simulink model "EHB_MOTOR"  (R2023b)
settings: Solver=FixedStepDiscrete  StartTime=0.0  StopTime=inf  FixedStep=0.0001  RelTol=1e-3  EnableMultiTasking=on
undefined symbols (not defined in the file): CAN_EHB_VCU0x125, CAN_EHB_VCU0x126, CAN_id0x120_Data, Cos_Table, Cos_Table1, EHB_DTC_status, R, Sin_BreakPoint, Sin_BreakPoint1, Sin_Table, Sin_Table1, T
libraries: simulink x30
(part 1 of 9)
settings Model: Creator=dell  LastModifiedBy=17802
settings SolverCC: AlgebraicLoopSolver=TrustRegion  PositivePriorityOrder=on  AutoInsertRateTranBlk=on
settings DataIOCC: LimitDataPoints=on  ReturnWorkspaceOutputs=off
settings OptimizationCC: DefaultParameterBehavior=Inlined  UseDivisionForNetSlopeComputation=on  GainParamInheritBuiltInType=on  UseFloatMulNetSlope=on  InlineInvariantSignals=on  PassReuseOutputArgsAs=Individual arguments  ExpressionDepthLimit=2147483647  ZeroExternalMemoryAtStartup=off  ZeroInternalMemoryAtStartup=off  NoFixptDivByZeroProtection=on  EfficientFloat2IntCast=on  LifeSpan=1  MaxStackSize=64  EfficientTunableParamExpr=on
settings DebuggingCC: CheckSSInitialOutputMsg=off  UnderspecifiedInitializationDetection=Classic  MergeDetectMultiDrivingBlocksExec=none  SolverPrmCheckMsg=warning  ParameterOverflowMsg=none  ParameterPrecisionLossMsg=none  FcnCallInpInsideContextMsg=warning  UnconnectedInputMsg=warning  UnconnectedOutputMsg=warning  UnconnectedLineMsg=warning  AssertControl=EnableAll  StateNameClashWarn=warning  SFUnexpectedBacktrackingDiag=warning  SFNoUnconditionalDefaultTransitionDiag=warning  SFExecutionAtInitializationDiag=none  ArithmeticOperatorsInVariantConditions=warning
settings HardwareCC: ProdBitPerPointer=32  ProdBitPerSizeT=32  ProdBitPerPtrDiffT=32  ProdLargestAtomicInteger=Long  ProdLargestAtomicFloat=Double  ProdEndianess=BigEndian  ProdWordSize=32  ProdHWDeviceType=Freescale->MPC5xx  TargetLargestAtomicInteger=Long  TargetLargestAtomicFloat=Double  TargetIntDivRoundTo=Zero  TargetEndianess=BigEndian  TargetHWDeviceType=Freescale->32-bit PowerPC  ProdEqTarget=off
settings ModelReferenceCC: UpdateModelReferenceTargets=IfOutOfDate  EnableRefExpFcnMdlSchedulingChecks=on  PropagateSignalLabelsOutOfModel=off
settings SFSimCC: SimUseLocalCustomCode=off  MATLABDynamicMemAlloc=off  CustomCodeUndefinedFunction=UseInterfaceOnly
settings SFSimCC: SimCustomHeaderCode=|
  | #define MCU_IDLE_ST     0
  | #define MCU_INIT_ST     1
  | #define MCU_START_ST    2
  | #define MCU_RUN_ST      3
  | #define MCU_FAULT_ST    4
  | #define MCU_WAIT_ST     5
  | 
  | // MCU_IDLE_ST = 0;
  | // MCU_INIT_ST = 1;
  | // MCU_START_ST = 2;
  | // MCU_RUN_ST = 3;
  | // MCU_FAULT_ST = 4;
  | // MCU_WAIT_ST = 5;
settings RTWCC: Description=Embedded Coder  SystemTargetFile=ert.tlc  GenCodeOnly=on  TemplateMakefile=ert_default_tmf  RTWUseLocalCustomCode=off  RTWUseSimCustomCode=on  IncludeHyperlinkInReport=on
settings RTWCC: CustomHeaderCode=|
  | #define MCU_IDLE_ST     0
  | #define MCU_INIT_ST     1
  | #define MCU_START_ST    2
  | #define MCU_RUN_ST      3
  | #define MCU_FAULT_ST    4
  | #define MCU_WAIT_ST     5
  | 
  | // MCU_IDLE_ST = 0;
  | // MCU_INIT_ST = 1;
  | // MCU_START_ST = 2;
  | // MCU_RUN_ST = 3;
  | // MCU_FAULT_ST = 4;
  | // MCU_WAIT_ST = 5;
settings CodeAppCC: ForceParamTrailComments=on  IgnoreCustomStorageClasses=off  SimulinkDataObjDesc=on  CustomSymbolStrGlobalVar=EHB_MOTOR_$N$M  CustomSymbolStrType=$N$M  CustomSymbolStrFcn=$N$M$F  CustomSymbolStrFcnArg=EHB_MOTOR_$I$N$M  CustomSymbolStrBlkIO=EHB_MOTOR_B_$N$M  CustomSymbolStrMacro=$N$M  InsertBlockDesc=on  InternalIdentifier=Classic
settings ERTTargetCC: MultiwordLength=2048  IncludeMdlTerminateFcn=off  CombineSignalStateStructs=on  IncludeFileDelimiter=UseQuote  SupportAbsoluteTime=off  SupportComplex=off  SupportNonInlinedSFcns=on  InlinedParameterPlacement=NonHierarchical  ERTCustomFileTemplate=example_file_process.tlc  GlobalDataDefinition=InSeparateSourceFile  DataDefinitionFile=EHB_MOTOR_data.c  GlobalDataReference=InSeparateHeaderFile  ERTFilePackagingFormat=CompactWithDataFile  DataReferenceFile=EHB_MOTOR.h  ConvertIfToSwitch=off  SuppressUnreachableDefaultCases=off  IndentStyle=Allman  IndentSize=4  MemSecPackage=mpt
settings ConfigComp: CovMetricSettings=dw  CovSaveCumulativeToWorkspaceVar=on  CovSaveSingleToWorkspaceVar=on  CovExternalEMLEnable=off  CovSFcnEnable=off
settings SimscapeCC: SimscapeNormalizeSystem=off
settings ConfigurationSet: Description=SimMechanics 2G

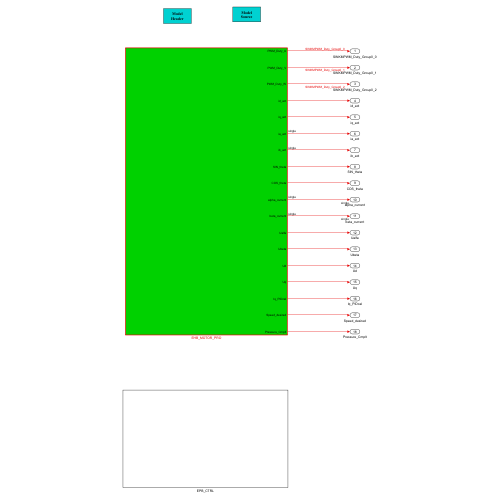
[thumbnail: Simulink's stored preview of the top-level diagram]
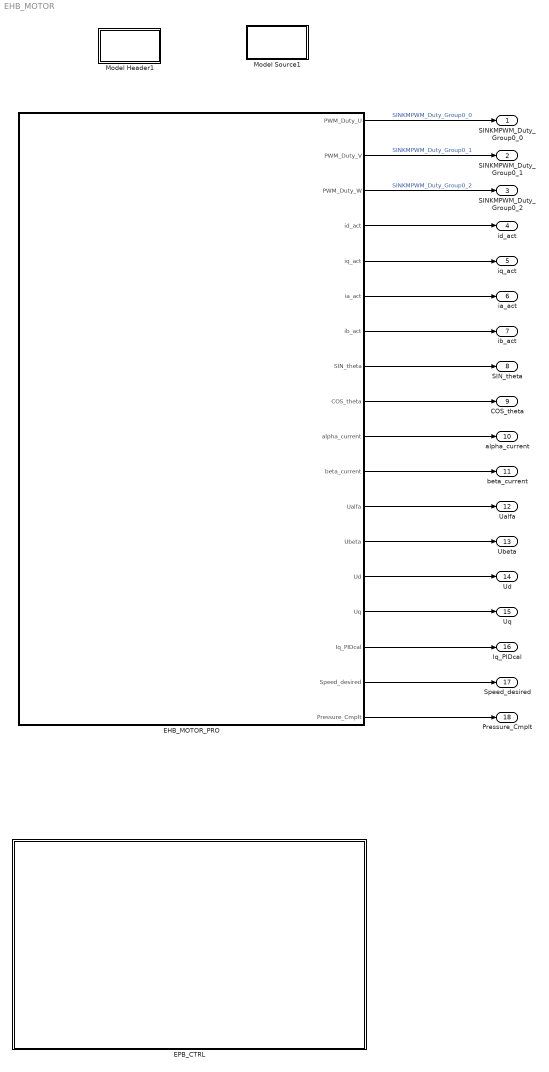
== system EHB_MOTOR ==
  EHB_MOTOR_PRO : Subsystem  TreatAsAtomicUnit=on  RTWFcnName=isr_can_rx
      settings: MinAlgLoopOccurrences=on
  EPB_CTRL : Subsystem
  Model Header1 : Subsystem  mask(Model Header){ShowInLibBrowser=0}
      mask prompts: ShowInLibBrowser "Simulink:masks:CustCodeMaskParam1_MP"
      settings: CopyFcn=cccopyfcn(gcb)  OpenFcn=ccopenfcn('Model Header')
      mask Help: eval('feval(''rtwprivate'',''rtwhelpview'',''rtw_model_header_block'')');
      mask Display: disp('Model\nHeader');
  Model Source1 : Subsystem  mask(Model Source){ShowInLibBrowser=0}
      mask prompts: ShowInLibBrowser "Simulink:masks:CustCodeMaskParam1_MP"
      settings: CopyFcn=cccopyfcn(gcb)  OpenFcn=ccopenfcn('Model Source')
      mask Help: eval('feval(''rtwprivate'',''rtwhelpview'',''rtw_model_source_block'')');
      mask Display: disp('Model\nSource');
  SINKMPWM_Duty_Group0_0 : Outport  VectorParamsAs1DForOutWhenUnconnected=off
  SINKMPWM_Duty_Group0_1 : Outport  Port=2  VectorParamsAs1DForOutWhenUnconnected=off
  SINKMPWM_Duty_Group0_2 : Outport  Port=3  VectorParamsAs1DForOutWhenUnconnected=off
  id_act : Outport  Port=4  VectorParamsAs1DForOutWhenUnconnected=off
  iq_act : Outport  Port=5  VectorParamsAs1DForOutWhenUnconnected=off
  ia_act : Outport  Port=6  VectorParamsAs1DForOutWhenUnconnected=off
  ib_act : Outport  Port=7  VectorParamsAs1DForOutWhenUnconnected=off
  SIN_theta : Outport  Port=8  VectorParamsAs1DForOutWhenUnconnected=off
  COS_theta : Outport  Port=9  VectorParamsAs1DForOutWhenUnconnected=off
  alpha_current : Outport  Port=10  OutDataTypeStr=single  VectorParamsAs1DForOutWhenUnconnected=off
  beta_current : Outport  Port=11  OutDataTypeStr=single  VectorParamsAs1DForOutWhenUnconnected=off
  Ualfa : Outport  Port=12  VectorParamsAs1DForOutWhenUnconnected=off
  Ubeta : Outport  Port=13  VectorParamsAs1DForOutWhenUnconnected=off
  Ud : Outport  Port=14  VectorParamsAs1DForOutWhenUnconnected=off
  Uq : Outport  Port=15  VectorParamsAs1DForOutWhenUnconnected=off
  Iq_PIDcal : Outport  Port=16  VectorParamsAs1DForOutWhenUnconnected=off
  Speed_desired : Outport  Port=17  VectorParamsAs1DForOutWhenUnconnected=off
  Pressure_Cmplt : Outport  Port=18  VectorParamsAs1DForOutWhenUnconnected=off
  wires:
  EHB_MOTOR_PRO/18(Pressure_Cmplt) -> Pressure_Cmplt/1
  EHB_MOTOR_PRO/4(id_act) -> id_act/1
  EHB_MOTOR_PRO/7(ib_act) -> ib_act/1
  EHB_MOTOR_PRO/16(Iq_PIDcal) -> Iq_PIDcal/1
  EHB_MOTOR_PRO/11(beta_current) -> beta_current/1
  EHB_MOTOR_PRO/15(Uq) -> Uq/1
  EHB_MOTOR_PRO/5(iq_act) -> iq_act/1
  EHB_MOTOR_PRO/13(Ubeta) -> Ubeta/1
  EHB_MOTOR_PRO/3(PWM_Duty_W) -> SINKMPWM_Duty_Group0_2/1  "SINKMPWM_Duty_Group0_2"
  EHB_MOTOR_PRO/17(Speed_desired) -> Speed_desired/1
  EHB_MOTOR_PRO/8(SIN_theta) -> SIN_theta/1
  EHB_MOTOR_PRO/6(ia_act) -> ia_act/1
  EHB_MOTOR_PRO/9(COS_theta) -> COS_theta/1
  EHB_MOTOR_PRO/14(Ud) -> Ud/1
  EHB_MOTOR_PRO/10(alpha_current) -> alpha_current/1
  EHB_MOTOR_PRO/2(PWM_Duty_V) -> SINKMPWM_Duty_Group0_1/1  "SINKMPWM_Duty_Group0_1"
  EHB_MOTOR_PRO/12(Ualfa) -> Ualfa/1
  EHB_MOTOR_PRO/1(PWM_Duty_U) -> SINKMPWM_Duty_Group0_0/1  "SINKMPWM_Duty_Group0_0"

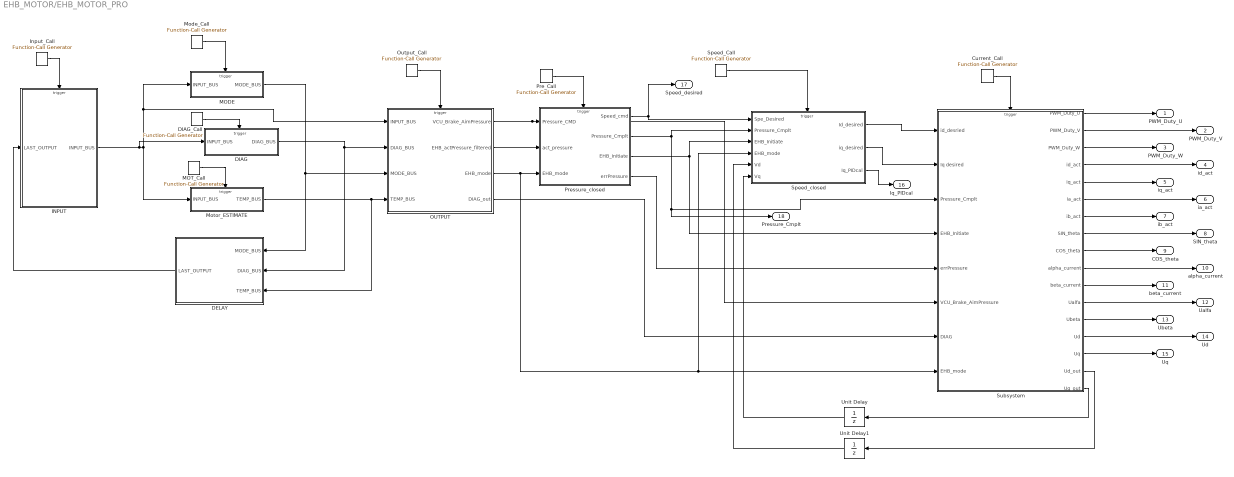
== system EHB_MOTOR/EHB_MOTOR_PRO ==
  Current_Call : simulink/Ports & Subsystems/Function-Call Generator  sample_time=0.0001  numberOfIterations=1  DisallowWideOutput=off
  DELAY : Subsystem
  DIAG : Subsystem
  DIAG_Call : simulink/Ports & Subsystems/Function-Call Generator  sample_time=0.01  numberOfIterations=1  DisallowWideOutput=off
  INPUT : Subsystem
  "Input_Call " : simulink/Ports & Subsystems/Function-Call Generator  sample_time=0.01  numberOfIterations=1  DisallowWideOutput=off
  MODE : Subsystem
  MOT_Call : simulink/Ports & Subsystems/Function-Call Generator  sample_time=0.01  numberOfIterations=1  DisallowWideOutput=off
  Mode_Call : simulink/Ports & Subsystems/Function-Call Generator  sample_time=0.01  numberOfIterations=1  DisallowWideOutput=off
  Motor_ESTIMATE : Subsystem
  OUTPUT : Subsystem
  Output_Call : simulink/Ports & Subsystems/Function-Call Generator  sample_time=0.01  numberOfIterations=1  DisallowWideOutput=off
  Pre_Call : simulink/Ports & Subsystems/Function-Call Generator  sample_time=0.002  numberOfIterations=1  DisallowWideOutput=off
  Pressure_closed : Subsystem
  "Speed_Call " : simulink/Ports & Subsystems/Function-Call Generator  sample_time=0.001  numberOfIterations=1  DisallowWideOutput=off
  Speed_closed : Subsystem
  Subsystem : Subsystem
  Unit Delay : UnitDelay  SampleTime=-1  HasFrameUpgradeWarning=on
  Unit Delay1 : UnitDelay  SampleTime=-1  HasFrameUpgradeWarning=on
  PWM_Duty_U : Outport  VectorParamsAs1DForOutWhenUnconnected=off
  PWM_Duty_V : Outport  Port=2  VectorParamsAs1DForOutWhenUnconnected=off
  PWM_Duty_W : Outport  Port=3  VectorParamsAs1DForOutWhenUnconnected=off
  id_act : Outport  Port=4  VectorParamsAs1DForOutWhenUnconnected=off
  iq_act : Outport  Port=5  VectorParamsAs1DForOutWhenUnconnected=off
  ia_act : Outport  Port=6  OutDataTypeStr=single  VectorParamsAs1DForOutWhenUnconnected=off
  ib_act : Outport  Port=7  OutDataTypeStr=single  VectorParamsAs1DForOutWhenUnconnected=off
  SIN_theta : Outport  Port=8  VectorParamsAs1DForOutWhenUnconnected=off
  COS_theta : Outport  Port=9  VectorParamsAs1DForOutWhenUnconnected=off
  alpha_current : Outport  Port=10  OutDataTypeStr=single  VectorParamsAs1DForOutWhenUnconnected=off
  beta_current : Outport  Port=11  OutDataTypeStr=single  VectorParamsAs1DForOutWhenUnconnected=off
  Ualfa : Outport  Port=12  VectorParamsAs1DForOutWhenUnconnected=off
  Ubeta : Outport  Port=13  VectorParamsAs1DForOutWhenUnconnected=off
  Ud : Outport  Port=14  VectorParamsAs1DForOutWhenUnconnected=off
  Uq : Outport  Port=15  VectorParamsAs1DForOutWhenUnconnected=off
  Iq_PIDcal : Outport  Port=16  VectorParamsAs1DForOutWhenUnconnected=off
  Speed_desired : Outport  Port=17  VectorParamsAs1DForOutWhenUnconnected=off
  Pressure_Cmplt : Outport  Port=18  VectorParamsAs1DForOutWhenUnconnected=off
  wires:
  "Speed_Call "/1 -> Speed_closed/Trigger
  Pressure_closed/1(Speed_cmd) -> Speed_closed/1(Spe_Desired), Speed_desired/1
  Subsystem/1(PWM_Duty_U) -> PWM_Duty_U/1
  Subsystem/2(PWM_Duty_V) -> PWM_Duty_V/1
  Subsystem/3(PWM_Duty_W) -> PWM_Duty_W/1
  Subsystem/4(id_act) -> id_act/1
  Subsystem/5(iq_act) -> iq_act/1
  Subsystem/6(ia_act) -> ia_act/1
  Subsystem/7(ib_act) -> ib_act/1
  Subsystem/8(SIN_theta) -> SIN_theta/1
  Subsystem/9(COS_theta) -> COS_theta/1
  Subsystem/10(alpha_current) -> alpha_current/1
  Subsystem/11(beta_current) -> beta_current/1
  Subsystem/12(Ualfa) -> Ualfa/1
  Subsystem/13(Ubeta) -> Ubeta/1
  Subsystem/14(Ud) -> Ud/1
  Subsystem/15(Uq) -> Uq/1
  Current_Call/1 -> Subsystem/Trigger
  OUTPUT/1(VCU_Brake_AimPressure) -> Pressure_closed/1(Pressure_CMD), Subsystem/6(VCU_Brake_AimPressure)
  Pressure_closed/4(errPressure) -> Subsystem/5(errPressure)
  Pressure_closed/2(Pressure_Cmplt) -> Speed_closed/2(Pressure_Cmplt), Pressure_Cmplt/1, Subsystem/3(Pressure_Cmplt)
  OUTPUT/4(DIAG_out) -> Subsystem/7(DIAG)
  Pressure_closed/3(EHB_Initiate) -> Speed_closed/3(EHB_Initiate), Subsystem/4(EHB_Initiate)
  Pre_Call/1 -> Pressure_closed/Trigger
  "Input_Call "/1 -> INPUT/Trigger
  DIAG/1(DIAG_BUS) -> DELAY/2(DIAG_BUS), OUTPUT/2(DIAG_BUS)
  Motor_ESTIMATE/1(TEMP_BUS) -> DELAY/3(TEMP_BUS), OUTPUT/4(TEMP_BUS)
  MODE/1(MODE_BUS) -> DELAY/1(MODE_BUS), OUTPUT/3(MODE_BUS)
  DELAY/1(LAST_OUTPUT) -> INPUT/1(LAST_OUTPUT)
  OUTPUT/2(EHB_actPressure_filtered) -> Pressure_closed/2(act_pressure)
  INPUT/1(INPUT_BUS) -> Motor_ESTIMATE/1(INPUT_BUS), MODE/1(INPUT_BUS), OUTPUT/1(INPUT_BUS), DIAG/1(INPUT_BUS)
  Speed_closed/1(Id_desired) -> Subsystem/1(id_desried)
  Mode_Call/1 -> MODE/Trigger
  DIAG_Call/1 -> DIAG/Trigger
  Output_Call/1 -> OUTPUT/Trigger
  MOT_Call/1 -> Motor_ESTIMATE/Trigger
  OUTPUT/3(EHB_mode) -> Pressure_closed/3(EHB_mode), Speed_closed/4(EHB_mode), Subsystem/8(EHB_mode)
  Subsystem/17(Uq_out) -> Unit Delay/1
  Subsystem/16(Ud_out) -> Unit Delay1/1
  Unit Delay/1 -> Speed_closed/6(Vq)
  Unit Delay1/1 -> Speed_closed/5(Vd)
  Speed_closed/2(iq_desired) -> Subsystem/2(Iq desired)
  Speed_closed/3(Iq_PIDcal) -> Iq_PIDcal/1

== system EHB_MOTOR/EPB_CTRL ==
  Data Store Memory : DataStoreMemory  DataStoreName=EPB_PWMout  ReadBeforeWriteMsg=warning  WriteAfterWriteMsg=warning  WriteAfterReadMsg=warning  ShowAdditionalParam=off  OutDataTypeStr=uint16
  Data Store Memory1 : DataStoreMemory  DataStoreName=EPB_state  ReadBeforeWriteMsg=warning  WriteAfterWriteMsg=warning  WriteAfterReadMsg=warning  ShowAdditionalParam=off  OutDataTypeStr=uint8
  Data Store Memory2 : DataStoreMemory  DataStoreName=EPB_CMD  ReadBeforeWriteMsg=warning  WriteAfterWriteMsg=warning  WriteAfterReadMsg=warning  ShowAdditionalParam=off  OutDataTypeStr=uint8
  Data Store Memory3 : DataStoreMemory  DataStoreName=Clamp_ok  ReadBeforeWriteMsg=warning  WriteAfterWriteMsg=warning  WriteAfterReadMsg=warning  ShowAdditionalParam=off  OutDataTypeStr=boolean
  Data Store Memory4 : DataStoreMemory  DataStoreName=Release_ok  ReadBeforeWriteMsg=warning  WriteAfterWriteMsg=warning  WriteAfterReadMsg=warning  ShowAdditionalParam=off  OutDataTypeStr=boolean
  Data Store Read : DataStoreRead  DataStoreName=EPB_CMD  DataStoreElements=EPB_CMD  IndexOptions=Index vector (dialog)  Indices=1  OutputSizes=1
  Data Store Write : DataStoreWrite  DataStoreName=EPB_PWMout  DataStoreElements=EPB_PWMout  IndexOptions=Index vector (dialog)  Indices=1  OutputSizes=1
  Data Store Write1 : DataStoreWrite  DataStoreName=EPB_state  DataStoreElements=EPB_state  IndexOptions=Index vector (dialog)  Indices=1  OutputSizes=1
  Data Store Write2 : DataStoreWrite  DataStoreName=Clamp_ok  DataStoreElements=Clamp_ok  IndexOptions=Index vector (dialog)  Indices=1  OutputSizes=1
  Data Store Write3 : DataStoreWrite  DataStoreName=Release_ok  DataStoreElements=Release_ok  IndexOptions=Index vector (dialog)  Indices=1  OutputSizes=1
  EPBDiag_Call : simulink/Ports & Subsystems/Function-Call Generator  sample_time=0.02  numberOfIterations=1  DisallowWideOutput=off
  EPBInput_Call : simulink/Ports & Subsystems/Function-Call Generator  sample_time=0.02  numberOfIterations=1  DisallowWideOutput=off
  EPB_CTRL : Subsystem
  EPB_Diag : Subsystem
  EPBctrl_Call : simulink/Ports & Subsystems/Function-Call Generator  sample_time=0.02  numberOfIterations=1  DisallowWideOutput=off
  Subsystem1 : Subsystem
  wires:
  EPB_Diag/1(EPB_DiagBUS) -> EPB_CTRL/2(EPB_DiagBUS)
  Subsystem1/1(EPB_INPUTBUS) -> EPB_Diag/1(In1), EPB_CTRL/3(EPB_INPUTBUS)
  EPBInput_Call/1 -> Subsystem1/Trigger
  EPB_CTRL/2(EPB_state) -> Data Store Write1/1
  EPB_CTRL/4(Release_ok) -> Data Store Write3/1
  EPBctrl_Call/1 -> EPB_CTRL/Trigger
  EPB_CTRL/1(EPB_PWMout) -> Data Store Write/1
  Data Store Read/1 -> EPB_CTRL/1(EPB_CMD)
  EPB_CTRL/3(Clamp_ok) -> Data Store Write2/1
  EPBDiag_Call/1 -> EPB_Diag/Trigger

== system EHB_MOTOR/Model Header1 ==

== system EHB_MOTOR/Model Source1 ==

== system EHB_MOTOR/EHB_MOTOR_PRO/DELAY ==
  MODE_BUS : Inport
  DIAG_BUS : Inport  Port=2
  TEMP_BUS : Inport  Port=3
  Bus Creator : BusCreator  Inputs=3
  Unit Delay : UnitDelay  SampleTime=-1  HasFrameUpgradeWarning=on
  Unit Delay1 : UnitDelay  SampleTime=-1  HasFrameUpgradeWarning=on
  Unit Delay2 : UnitDelay  SampleTime=-1  HasFrameUpgradeWarning=on
  LAST_OUTPUT : Outport  VectorParamsAs1DForOutWhenUnconnected=off
  wires:
  MODE_BUS/1 -> Unit Delay/1
  DIAG_BUS/1 -> Unit Delay1/1
  Unit Delay/1 -> Bus Creator/1  "MODE_DELAY"
  Unit Delay1/1 -> Bus Creator/2  "DIAG_DELAY"
  Unit Delay2/1 -> Bus Creator/3  "TEMP_DELAY"
  Bus Creator/1 -> LAST_OUTPUT/1
  TEMP_BUS/1 -> Unit Delay2/1

== system EHB_MOTOR/EHB_MOTOR_PRO/DIAG ==
  INPUT_BUS : Inport
  Trigger : TriggerPort  TriggerType=function-call  VariantControl=Variant  PortDimensions=1
  5vDiag : Subsystem
  AngleSensorDiag : Subsystem
  Bus Creator : BusCreator  Inputs=24
  Bus Selector : BusSelector  OutputSignals=MOT_BUS.Motor_Angle
  Bus Selector1 : BusSelector  OutputSignals=CAN_BUS.VCU_Brake_AimPressure,AI_BUS.EHB_actPresure_filtered,AI_BUS.EHB_Presure_ADC
  Bus Selector10 : BusSelector  OutputSignals=AI_BUS.EHB_5vOUT_filtered
  Bus Selector14 : BusSelector  OutputSignals=AI_BUS.EHB_vWheel_filtered
  Bus Selector4 : BusSelector  OutputSignals=AI_BUS.EHB_vBAT_filtered
  Bus Selector6 : BusSelector  OutputSignals=AI_BUS.EHB_12vLogic_filtered
  Bus Selector7 : BusSelector  OutputSignals=AI_BUS.EHB_vKL15_filtered
  Bus Selector8 : BusSelector  OutputSignals=AI_BUS.EHB_iU_filtered,AI_BUS.EHB_iV_filtered,AI_BUS.EHB_iW_filtered
  Bus Selector9 : BusSelector  OutputSignals=AI_BUS.EHB_Temp
  BusOffDiag : Subsystem  Commented=on
  CANCommDiag : Subsystem  Commented=on
  CANDataLostDiag : Subsystem  Commented=on
  Chip7189Diag : Subsystem
  CurrentSensorDiag : Subsystem
  DIAG_OUT : Subsystem
  Data Store Memory : DataStoreMemory  DataStoreName=EHB_DTC_status  ReadBeforeWriteMsg=warning  WriteAfterWriteMsg=warning  WriteAfterReadMsg=warning  ShowAdditionalParam=off  OutDataTypeStr=uint8  Dimensions=50
  Data Store Write : DataStoreWrite  DataStoreName=EHB_DTC_status  DataStoreElements=EHB_DTC_status(:)  IndexOptions=Index vector (dialog)  Indices=1  OutputSizes=1
  EHBDiag : Subsystem
  Ground : Ground
  Ground1 : Ground
  KL15VoltageDiag : Subsystem
  LogicVoltageDiag : Subsystem
  MotLockDiag : Subsystem
  MotorDiag : Subsystem  Commented=on
  PWMCircuitDiag : Subsystem  Commented=on
  PressureSensorDiag : Subsystem
  RespondOvertimeDiag : Subsystem  Commented=on
  SpeedSensorDiag : Subsystem
  TLF35584Diag : Subsystem
  TempDiag : Subsystem
  UDS_interface : Subsystem
  DIAG_BUS : Outport  VectorParamsAs1DForOutWhenUnconnected=off
  wires:
  Bus Creator/1 -> DIAG_OUT/1(DIAG_BUS), DIAG_BUS/1, UDS_interface/1(DiagBUS)
  INPUT_BUS/1 -> Bus Selector14/1, MotLockDiag/1(In1), Bus Selector10/1, Bus Selector9/1, Bus Selector8/1, Bus Selector7/1, Bus Selector6/1, Bus Selector4/1, Bus Selector1/1, Bus Selector/1
  AngleSensorDiag/1(AngleSensorSignalOverride) -> Bus Creator/1  "AngleSensorSignalOverride"
  AngleSensorDiag/2(AngleSensorSignalLost) -> Bus Creator/2  "AngleSensorSignalLost"
  AngleSensorDiag/3(AngleSensorNoCal) -> Bus Creator/3  "AngleSensorNoCal"
  PressureSensorDiag/1(PressureFlowERR1) -> Bus Creator/4  "PressureFlowERR1"
  PressureSensorDiag/3(PressureSensorERR) -> Bus Creator/6  "PressureSensorERR"
  PressureSensorDiag/4(PressureSensorNoCal) -> Bus Creator/7  "PressureSensorNoCal"
  Bus Selector/1 -> AngleSensorDiag/1(AngleSensorSignal)  "<Motor_Angle>"
  Bus Selector1/2 -> PressureSensorDiag/2(EHB_actPresure_filtered)  "<EHB_actPresure_filtered>"
  EHBDiag/1(EHBVoltageLow1) -> Bus Creator/8  "EHBVoltageLow1"
  EHBDiag/3(EHBVoltageHigh1) -> Bus Creator/10  "EHBVoltageHigh1"
  Bus Selector4/1 -> EHBDiag/1(EHBVoltage)  "<EHB_vBAT_filtered>"
  LogicVoltageDiag/1(LogicVoltageLow) -> Bus Creator/12  "LogicVoltageLow"
  LogicVoltageDiag/2(LogicVoltageHigh) -> Bus Creator/13  "LogicVoltageHigh"
  Bus Selector6/1 -> LogicVoltageDiag/1(LogicVoltage)  "<EHB_12vLogic_filtered>"
  KL15VoltageDiag/1(KL15VoltageLow) -> Bus Creator/14  "KL15VoltageLow"
  KL15VoltageDiag/2(KL15VoltageHigh) -> Bus Creator/15  "KL15VoltageHigh"
  Bus Selector7/1 -> KL15VoltageDiag/1(KL15Voltage)  "<EHB_vKL15_filtered>"
  CurrentSensorDiag/1(CurrentSensorUOverride) -> Bus Creator/16  "CurrentSensorUOverride"
  CurrentSensorDiag/2(CurrentSensorVOverride) -> Bus Creator/17  "CurrentSensorVOverride"
  CurrentSensorDiag/3(CurrentSensorWOverride) -> Bus Creator/18  "CurrentSensorWOverride"
  Bus Selector8/1 -> CurrentSensorDiag/1(CurrentSensorU)  "<EHB_iU_filtered>"
  Bus Selector8/2 -> CurrentSensorDiag/2(CurrentSensorV)  "<EHB_iV_filtered>"
  TempDiag/1(TempSensorOverride) -> Bus Creator/19  "TempSensorOverride"
  Bus Selector9/1 -> TempDiag/1(TempSensor)  "<EHB_Temp>"
  Bus Selector10/1 -> 5vDiag/1(5vVoltage)  "<EHB_5vOUT_filtered>"
  5vDiag/1(5vErr) -> Bus Creator/20  "5vErr"
  Chip7189Diag/1(Chip7189_err) -> Bus Creator/21  "Chip7189_err"
  SpeedSensorDiag/1(SpeedSensorOverride) -> Bus Creator/22  "SpeedSensorOverride"
  Bus Selector14/1 -> SpeedSensorDiag/1(SpeedSensor)  "<EHB_vWheel_filtered>"
  Ground/1 -> AngleSensorDiag/2(AngleSensorCalFlag)
  Ground1/1 -> PressureSensorDiag/4(PressureSensorCalFlag)
  Bus Selector8/3 -> CurrentSensorDiag/3(CurrentSensorW)  "<EHB_iW_filtered>"
  Bus Selector1/1 -> PressureSensorDiag/1(VCU_Brake_AimPressure)  "<VCU_Brake_AimPressure>"
  PressureSensorDiag/2(PressureFlowERR2) -> Bus Creator/5  "PressureFlowERR2"
  EHBDiag/2(EHBVoltageLow2) -> Bus Creator/9  "EHBVoltageLow2"
  EHBDiag/4(EHBVoltageHigh2) -> Bus Creator/11  "EHBVoltageHigh2"
  MotLockDiag/1(Mot_locked_err) -> Bus Creator/23  "Mot_locked_err"
  Bus Selector1/3 -> PressureSensorDiag/3(EHB_Presure_ADC)  "<EHB_Presure_ADC>"
  UDS_interface/1(EHB_DTC) -> Data Store Write/1
  TLF35584Diag/1(TLF35584err_BUS) -> Bus Creator/24  "TLF35584err_BUS"

== system EHB_MOTOR/EHB_MOTOR_PRO/INPUT ==
  LAST_OUTPUT : Inport
  Trigger : TriggerPort  TriggerType=function-call  VariantControl=Variant  PortDimensions=1
  AI : Subsystem
  Bus Creator : BusCreator  Inputs=5
  Bus Creator1 : BusCreator  Inputs=16
  Bus Creator2 : BusCreator  Inputs=5
  Bus Creator3 : BusCreator  Inputs=2
  Bus Creator4 : BusCreator  Inputs=10
  CAN : Subsystem
  DI : Subsystem
  MOTOR : Subsystem
  OUTPUT2INPUT : Subsystem
  INPUT_BUS : Outport  VectorParamsAs1DForOutWhenUnconnected=off
  wires:
  CAN/1(VCU_BrakingEnable) -> Bus Creator/1  "VCU_BrakingEnable"
  CAN/2(VCU_ParkingBrakeActive) -> Bus Creator/2  "VCU_ParkingBrakeActive"
  CAN/3(VCU_Brake_AimPressure) -> Bus Creator/3  "VCU_Brake_AimPressure"
  CAN/4(VCU_RollingCounter) -> Bus Creator/4  "VCU_RollingCounter"
  CAN/5(VCU_Checksum) -> Bus Creator/5  "VCU_Checksum"
  AI/1(EHB_vBAT_filtered) -> Bus Creator1/1  "EHB_vBAT_filtered"
  MOTOR/1(Motor_Angle) -> Bus Creator3/1  "Motor_Angle"
  Bus Creator/1 -> Bus Creator2/4  "CAN_BUS"
  AI/3(EHB_5vOUT_filtered) -> Bus Creator1/3  "EHB_5vOUT_filtered"
  MOTOR/2(Motor_actPWM) -> Bus Creator3/2  "Motor_actPWM"
  Bus Creator3/1 -> Bus Creator2/3  "MOT_BUS"
  LAST_OUTPUT/1 -> OUTPUT2INPUT/1(LAST_OUTPUT)
  AI/2(EHB_vKL15_filtered) -> Bus Creator1/2  "EHB_vKL15_filtered"
  AI/7(EHB_iU_filtered) -> Bus Creator1/7  "EHB_iU_filtered"
  AI/9(EHB_iV_filtered) -> Bus Creator1/9  "EHB_iV_filtered"
  AI/11(EHB_iW_filtered) -> Bus Creator1/11  "EHB_iW_filtered"
  AI/13(EHB_vWheel_filtered) -> Bus Creator1/13  "EHB_vWheel_filtered"
  DI/1(EHB_Ignion) -> Bus Creator4/1  "EHB_Ignion"
  DI/2(EHB_35584err1) -> Bus Creator4/2  "EHB_35584err1"
  DI/3(EHB_35584err2) -> Bus Creator4/3  "EHB_35584err2"
  DI/4(EHB_35584INT) -> Bus Creator4/4  "EHB_35584INT"
  DI/5(EHB_swBrkLED) -> Bus Creator4/5  "EHB_swBrkLED"
  DI/6(EHB_posLiq) -> Bus Creator4/6  "EHB_posLiq"
  DI/7(EHB_7189err1) -> Bus Creator4/7  "EHB_7189err1"
  DI/8(EHB_7189err2) -> Bus Creator4/8  "EHB_7189err2"
  DI/9(EHB_HID) -> Bus Creator4/9  "EHB_HID"
  DI/10(EHB_AVH) -> Bus Creator4/10  "EHB_AVH"
  Bus Creator4/1 -> Bus Creator2/2  "DI_BUS"
  AI/14(EHB_Reserve_filtered) -> Bus Creator1/14  "EHB_Reserve_filtered"
  AI/15(EHB_12vLogic_filtered) -> Bus Creator1/15  "EHB_12vLogic_filtered"
  AI/16(EHB_pwrPressure_filtered) -> Bus Creator1/16  "EHB_pwrPressure_filtered"
  OUTPUT2INPUT/1(Feedback) -> Bus Creator2/5  "Feedback"
  AI/8(EHB_iU_AD) -> Bus Creator1/8  "EHB_iU_AD"
  AI/10(EHB_iV_AD) -> Bus Creator1/10  "EHB_iV_AD"
  AI/12(EHB_iW_AD) -> Bus Creator1/12  "EHB_iW_AD"
  AI/5(EHB_Presure_ADC) -> Bus Creator1/5  "EHB_Presure_ADC"
  Bus Creator2/1 -> INPUT_BUS/1
  AI/4(EHB_Temp) -> Bus Creator1/4  "EHB_Temp"
  AI/6(EHB_actPresure_filtered) -> Bus Creator1/6  "EHB_actPresure_filtered"
  Bus Creator1/1 -> Bus Creator2/1  "AI_BUS"

== system EHB_MOTOR/EHB_MOTOR_PRO/MODE ==
  note: 待增加自检类故障
  INPUT_BUS : Inport
  Trigger : TriggerPort  TriggerType=function-call  VariantControl=Variant  PortDimensions=1
  Bus Creator : BusCreator  Inputs=9
  Bus Selector : BusSelector  OutputSignals=CAN_BUS.VCU_BrakingEnable
  Bus Selector1 : BusSelector  OutputSignals=AI_BUS.EHB_iU_AD,AI_BUS.EHB_iV_AD,AI_BUS.EHB_iW_AD
  Bus Selector2 : BusSelector  OutputSignals=MOT_BUS.Motor_Angle
  Bus Selector3 : BusSelector  OutputSignals=DI_BUS.EHB_Ignion
  Chart : Stateflow chart  TreatAsAtomicUnit=on
  Chart1 : Stateflow chart  TreatAsAtomicUnit=on
  Constant : Constant  OutDataTypeStr=uint8
  Constant1 : Constant  OutDataTypeStr=boolean
  Constant2 : Constant
  Constant3 : Constant
  Data Store Memory : DataStoreMemory  DataStoreName=ZeroCal_Flash_ok  ReadBeforeWriteMsg=warning  WriteAfterWriteMsg=warning  WriteAfterReadMsg=warning  ShowAdditionalParam=off  OutDataTypeStr=boolean
  Data Store Memory1 : DataStoreMemory  DataStoreName=Zero_Angle  ReadBeforeWriteMsg=warning  WriteAfterWriteMsg=warning  WriteAfterReadMsg=warning  ShowAdditionalParam=off  OutDataTypeStr=uint16
  Data Store Memory2 : DataStoreMemory  DataStoreName=ZeroCal_cmplt  ReadBeforeWriteMsg=warning  WriteAfterWriteMsg=warning  WriteAfterReadMsg=warning  ShowAdditionalParam=off  OutDataTypeStr=boolean
  Data Store Memory3 : DataStoreMemory  DataStoreName=ZeroCal_Req  ReadBeforeWriteMsg=warning  WriteAfterWriteMsg=warning  WriteAfterReadMsg=warning  ShowAdditionalParam=off  OutDataTypeStr=uint8
  Data Store Read : DataStoreRead  DataStoreName=ZeroCal_Flash_ok  DataStoreElements=ZeroCal_Flash_ok  IndexOptions=Index vector (dialog)  Indices=1  OutputSizes=1
  Data Store Write1 : DataStoreWrite  DataStoreName=Zero_Angle  DataStoreElements=Zero_Angle  IndexOptions=Index vector (dialog)  Indices=1  OutputSizes=1
  Data Store Write2 : DataStoreWrite  DataStoreName=ZeroCal_cmplt  DataStoreElements=ZeroCal_cmplt  IndexOptions=Index vector (dialog)  Indices=1  OutputSizes=1
  Data Store Write3 : DataStoreWrite  DataStoreName=ZeroCal_Req  DataStoreElements=ZeroCal_Req  IndexOptions=Index vector (dialog)  Indices=1  OutputSizes=1
  KL15_condition : Subsystem  Commented=on
  Relational Operator : RelationalOperator  Operator===  OutDataTypeStr=boolean  RndMeth=Simplest  InputSameDT=off
  Relational Operator1 : RelationalOperator  Operator===  OutDataTypeStr=boolean  RndMeth=Simplest  InputSameDT=off
  Subsystem : Subsystem
  Switch : Switch  Criteria=u2 ~= 0  SaturateOnIntegerOverflow=off  InputSameDT=off
  Unit Delay : UnitDelay  SampleTime=-1  HasFrameUpgradeWarning=on
  MODE_BUS : Outport  VectorParamsAs1DForOutWhenUnconnected=off
  wires:
  Bus Creator/1 -> MODE_BUS/1
  INPUT_BUS/1 -> Bus Selector3/1, Subsystem/1(INPUT_BUS), Bus Selector2/1, Bus Selector/1, Bus Selector1/1
  Bus Selector3/1 -> Chart/1(ignition)  "<EHB_Ignion>"
  Bus Selector/1 -> Chart/5(EHB_mode_req)  "<VCU_BrakingEnable>"
  Chart/1(EHB_35584_en) -> Bus Creator/1  "EHB_35584_en"
  Chart/2(EHB_5vOUT_en) -> Bus Creator/2  "EHB_5vOUT_en"
  Chart/3(EHB_7189_en) -> Bus Creator/3  "EHB_7189_en"
  Chart/4(EHB_CAN_en) -> Bus Creator/4  "EHB_CAN_en"
  Chart/5(EHB_mode) -> Bus Creator/5  "EHB_mode"
  Subsystem/1(Fault_Status) -> Chart/7(Fault_Sts)
  Bus Selector1/1 -> Chart/2(Motor_iUzero_AD)  "<EHB_iU_AD>"
  Bus Selector1/2 -> Chart/3(Motor_iVzero_AD)  "<EHB_iV_AD>"
  Bus Selector1/3 -> Chart/4(Motor_iWzero_AD)  "<EHB_iW_AD>"
  Chart/6(Flash_Ucurrent) -> Bus Creator/6  "Flash_Ucurrent"
  Chart/7(Flash_Vcurrent) -> Bus Creator/7  "Flash_Vcurrent"
  Chart/8(Flash_Wcurrent) -> Bus Creator/8  "Flash_Wcurrent"
  Chart/9(EHB_AngleZeroCal_Req) -> Bus Creator/9, Relational Operator/1, Data Store Write3/1  "EHB_AngleZeroCal_Req"
  Chart1/2(ZeroCal_cmplt) -> Data Store Write2/1, Unit Delay/1
  Constant/1 -> Chart/6(Self_Check_Sts)
  Relational Operator/1 -> Chart1/2(input)
  Constant2/1 -> Relational Operator/2
  Chart1/1(Zero_Angle) -> Data Store Write1/1
  Bus Selector2/1 -> Chart1/1(MOT_Angle)  "<Motor_Angle>"
  Unit Delay/1 -> Switch/3
  Switch/1 -> Chart/8(ZeroCal_write_ok)
  Constant1/1 -> Switch/1
  Relational Operator1/1 -> Switch/2
  Data Store Read/1 -> Relational Operator1/1
  Constant3/1 -> Relational Operator1/2

== system EHB_MOTOR/EHB_MOTOR_PRO/Motor_ESTIMATE ==
  INPUT_BUS : Inport
  Trigger : TriggerPort  TriggerType=function-call  VariantControl=Variant  PortDimensions=1
  Bus Creator : BusCreator  Inputs=2
  Bus Selector : BusSelector  OutputSignals=AI_BUS.EHB_Temp
  Bus Selector1 : BusSelector  OutputSignals=MOT_BUS.Motor_Angle
  Motor_Length : Subsystem
  Motor_Temp : Subsystem
  TEMP_BUS : Outport  VectorParamsAs1DForOutWhenUnconnected=off
  wires:
  Motor_Temp/1(EHB_Mot_temp) -> Bus Creator/1  "EHB_Mot_temp"
  Motor_Length/1(EHB_Mot_length) -> Bus Creator/2  "EHB_Mot_length"
  Bus Creator/1 -> TEMP_BUS/1
  INPUT_BUS/1 -> Bus Selector1/1, Bus Selector/1
  Bus Selector/1 -> Motor_Temp/1(In1)  "<EHB_Temp>"
  Bus Selector1/1 -> Motor_Length/1(In1)  "<Motor_Angle>"

== system EHB_MOTOR/EHB_MOTOR_PRO/OUTPUT ==
  INPUT_BUS : Inport
  DIAG_BUS : Inport  Port=2
  MODE_BUS : Inport  Port=3
  TEMP_BUS : Inport  Port=4
  Trigger : TriggerPort  TriggerType=function-call  VariantControl=Variant  PortDimensions=1
  CAN_pack : Subsystem
  Data Store Memory3 : DataStoreMemory  DataStoreName=CAN_EHB_VCU0x125  ReadBeforeWriteMsg=warning  WriteAfterWriteMsg=warning  WriteAfterReadMsg=warning  ShowAdditionalParam=off  OutDataTypeStr=uint8  Dimensions=8
  Data Store Memory4 : DataStoreMemory  DataStoreName=CAN_EHB_VCU0x126  ReadBeforeWriteMsg=warning  WriteAfterWriteMsg=warning  WriteAfterReadMsg=warning  ShowAdditionalParam=off  OutDataTypeStr=uint8  Dimensions=8
  Data Store Write2 : DataStoreWrite  DataStoreName=CAN_EHB_VCU0x125  DataStoreElements=CAN_EHB_VCU0x125(:)  IndexOptions=Index vector (dialog)  Indices=1  OutputSizes=1
  Data Store Write3 : DataStoreWrite  DataStoreName=CAN_EHB_VCU0x126  DataStoreElements=CAN_EHB_VCU0x126(:)  IndexOptions=Index vector (dialog)  Indices=1  OutputSizes=1
  FUALT_HANDLE : Subsystem
  VCU_Brake_AimPressure : Outport  VectorParamsAs1DForOutWhenUnconnected=off
  EHB_actPressure_filtered : Outport  Port=2  VectorParamsAs1DForOutWhenUnconnected=off
  EHB_mode : Outport  Port=3  VectorParamsAs1DForOutWhenUnconnected=off
  DIAG_out : Outport  Port=4  VectorParamsAs1DForOutWhenUnconnected=off
  wires:
  INPUT_BUS/1 -> FUALT_HANDLE/1(INPUT_BUS), CAN_pack/1(INPUT_BUS)
  FUALT_HANDLE/2(EHB_actPressure_filtered) -> EHB_actPressure_filtered/1
  DIAG_BUS/1 -> FUALT_HANDLE/3(DIAG_BUS), CAN_pack/3(DIAG_BUS)
  TEMP_BUS/1 -> FUALT_HANDLE/4(TEMP_BUS)
  MODE_BUS/1 -> FUALT_HANDLE/2(MODE_BUS), CAN_pack/2(MODE_BUS)
  FUALT_HANDLE/1(VCU_Brake_AimPressure) -> VCU_Brake_AimPressure/1
  CAN_pack/1(EHB_VCU_0x125) -> Data Store Write2/1
  CAN_pack/2(EHB_VCU_0x126) -> Data Store Write3/1
  FUALT_HANDLE/4(DIAG_out) -> DIAG_out/1
  FUALT_HANDLE/3(EHB_mode) -> EHB_mode/1

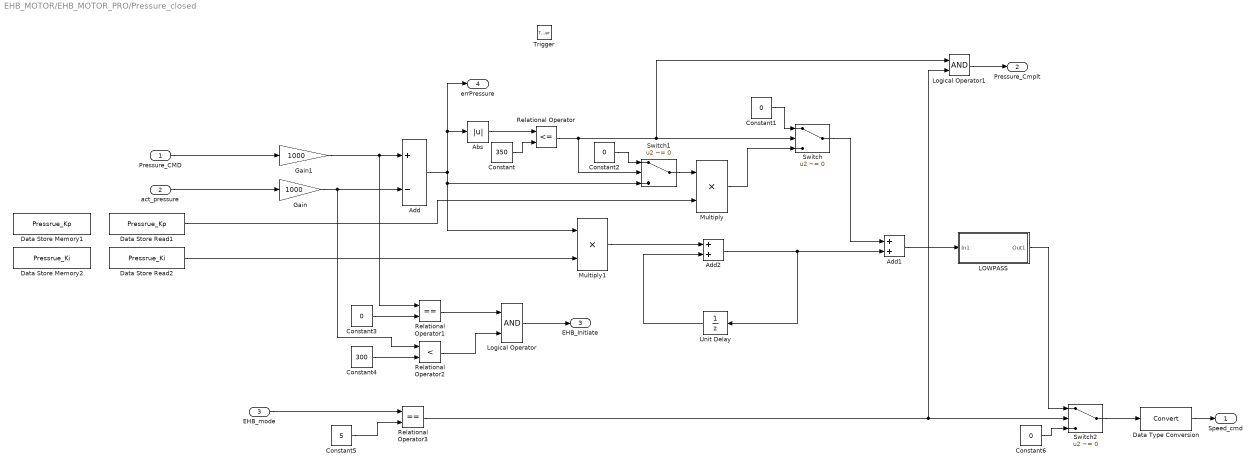
== system EHB_MOTOR/EHB_MOTOR_PRO/Pressure_closed ==
  Pressure_CMD : Inport
  act_pressure : Inport  Port=2
  EHB_mode : Inport  Port=3
  Trigger : TriggerPort  TriggerType=function-call  VariantControl=Variant  PortDimensions=1
  Abs : Abs  SaturateOnIntegerOverflow=off
  Add : Sum  Inputs=+-
  Add1 : Sum
  Add2 : Sum
  Constant : Constant  Value=350
  Constant1 : Constant  Value=0  OutDataTypeStr=single
  Constant2 : Constant  Value=0  OutDataTypeStr=single
  Constant3 : Constant  Value=0
  Constant4 : Constant  Value=300
  Constant5 : Constant  Value=5
  Constant6 : Constant  Value=0  OutDataTypeStr=single
  Data Store Memory1 : DataStoreMemory  DataStoreName=Pressrue_Kp  ReadBeforeWriteMsg=warning  WriteAfterWriteMsg=warning  WriteAfterReadMsg=warning  ShowAdditionalParam=off  OutDataTypeStr=single
  Data Store Memory2 : DataStoreMemory  DataStoreName=Pressrue_Ki  ReadBeforeWriteMsg=warning  WriteAfterWriteMsg=warning  WriteAfterReadMsg=warning  ShowAdditionalParam=off  OutDataTypeStr=single
  Data Store Read1 : DataStoreRead  DataStoreName=Pressrue_Kp  DataStoreElements=Pressrue_Kp  IndexOptions=Index vector (dialog)  Indices=1  OutputSizes=1
  Data Store Read2 : DataStoreRead  DataStoreName=Pressrue_Ki  DataStoreElements=Pressrue_Ki  IndexOptions=Index vector (dialog)  Indices=1  OutputSizes=1
  Data Type Conversion : DataTypeConversion  SaturateOnIntegerOverflow=off  RndMeth=Floor
  Gain : Gain  Gain=1000  OutDataTypeStr=single
  Gain1 : Gain  Gain=1000  OutDataTypeStr=single
  LOWPASS : Subsystem
  Logical Operator : Logic  AllPortsSameDT=off  OutDataTypeStr=boolean
  Logical Operator1 : Logic  AllPortsSameDT=off  OutDataTypeStr=boolean
  Multiply : Product
  Multiply1 : Product
  Relational Operator : RelationalOperator  Operator=<=  OutDataTypeStr=boolean  RndMeth=Simplest  InputSameDT=off
  Relational Operator1 : RelationalOperator  Operator===  OutDataTypeStr=boolean  RndMeth=Simplest  InputSameDT=off
  Relational Operator2 : RelationalOperator  Operator=<  OutDataTypeStr=boolean  RndMeth=Simplest  InputSameDT=off
  Relational Operator3 : RelationalOperator  Operator===  OutDataTypeStr=boolean  RndMeth=Simplest  InputSameDT=off
  Switch : Switch  Criteria=u2 ~= 0  SaturateOnIntegerOverflow=off  InputSameDT=off
  Switch1 : Switch  Criteria=u2 ~= 0  SaturateOnIntegerOverflow=off  InputSameDT=off
  Switch2 : Switch  Criteria=u2 ~= 0  SaturateOnIntegerOverflow=off  InputSameDT=off
  Unit Delay : UnitDelay  SampleTime=-1  HasFrameUpgradeWarning=on
  Speed_cmd : Outport  VectorParamsAs1DForOutWhenUnconnected=off
  Pressure_Cmplt : Outport  Port=2  VectorParamsAs1DForOutWhenUnconnected=off
  EHB_Initiate : Outport  Port=3  VectorParamsAs1DForOutWhenUnconnected=off
  errPressure : Outport  Port=4  VectorParamsAs1DForOutWhenUnconnected=off
  wires:
  Pressure_CMD/1 -> Gain1/1
  Gain1/1 -> Add/1, Relational Operator1/1
  Gain/1 -> Add/2, Relational Operator2/1
  Data Store Read1/1 -> Multiply/2
  Add1/1 -> LOWPASS/1(In1)
  Data Store Read2/1 -> Multiply1/2
  Multiply1/1 -> Add2/1
  Add2/1 -> Unit Delay/1, Add1/2
  Unit Delay/1 -> Add2/2
  Multiply/1 -> Switch/3
  Abs/1 -> Relational Operator/1
  Constant/1 -> Relational Operator/2
  Relational Operator/1 -> Logical Operator1/1, Switch/2, Switch1/2
  Switch/1 -> Add1/1
  Constant1/1 -> Switch/1
  LOWPASS/1(Out1) -> Switch2/1
  Switch1/1 -> Multiply/1
  Constant2/1 -> Switch1/1
  Add/1 -> Switch1/3, Multiply1/1, Abs/1, errPressure/1
  Constant3/1 -> Relational Operator1/2
  Constant4/1 -> Relational Operator2/2
  Relational Operator2/1 -> Logical Operator/2
  Relational Operator1/1 -> Logical Operator/1
  Logical Operator/1 -> EHB_Initiate/1
  act_pressure/1 -> Gain/1
  EHB_mode/1 -> Relational Operator3/1
  Constant5/1 -> Relational Operator3/2
  Relational Operator3/1 -> Switch2/2, Logical Operator1/2
  Switch2/1 -> Data Type Conversion/1
  Constant6/1 -> Switch2/3
  Logical Operator1/1 -> Pressure_Cmplt/1
  Data Type Conversion/1 -> Speed_cmd/1

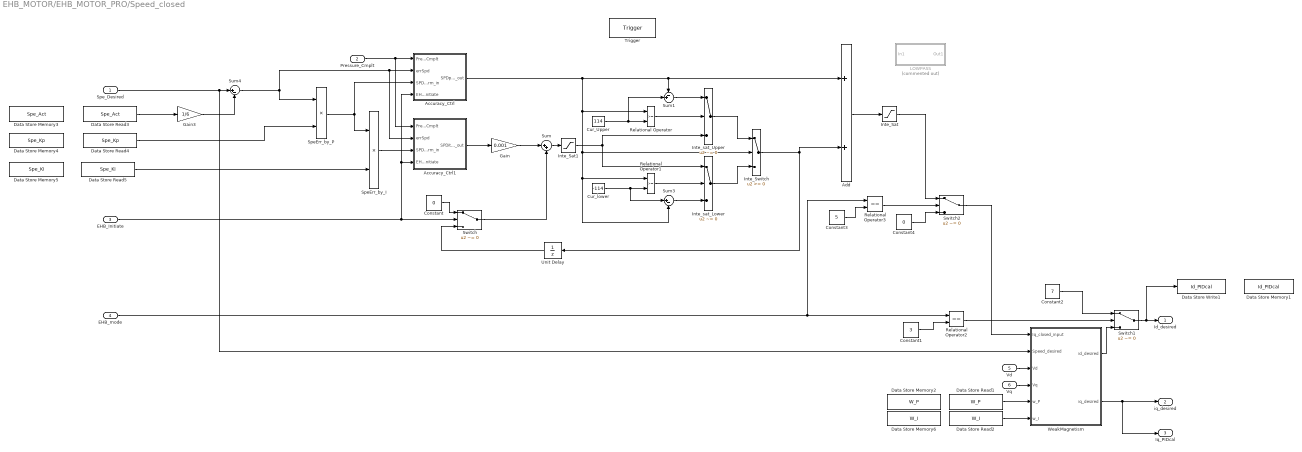
== system EHB_MOTOR/EHB_MOTOR_PRO/Speed_closed ==
  Spe_Desired : Inport  OutDataTypeStr=single
  Pressure_Cmplt : Inport  Port=2
  EHB_Initiate : Inport  Port=3
  EHB_mode : Inport  Port=4
  Vd : Inport  Port=5
  Vq : Inport  Port=6
  Trigger : TriggerPort  TriggerType=function-call  VariantControl=(inherit)  PortDimensions=1
  Accuracy_Ctrl : Subsystem
  Accuracy_Ctrl1 : Subsystem
  Add : Sum  OutDataTypeStr=single
  Constant : Constant  Value=0  OutDataTypeStr=single
  Constant1 : Constant  Value=3
  Constant2 : Constant  Value=7  OutDataTypeStr=single
  Constant3 : Constant  Value=5
  Constant4 : Constant  Value=0  OutDataTypeStr=single
  Cur_Upper : Constant  Value=114  OutDataTypeStr=single
  Cur_lower : Constant  Value=-114  OutDataTypeStr=single
  Data Store Memory1 : DataStoreMemory  DataStoreName=Id_PIDcal  ReadBeforeWriteMsg=warning  WriteAfterWriteMsg=warning  WriteAfterReadMsg=warning  ShowAdditionalParam=off  OutDataTypeStr=single
  Data Store Memory2 : DataStoreMemory  DataStoreName=W_P  ReadBeforeWriteMsg=warning  WriteAfterWriteMsg=warning  WriteAfterReadMsg=warning  ShowAdditionalParam=off  OutDataTypeStr=single
  Data Store Memory3 : DataStoreMemory  DataStoreName=Spe_Act  ReadBeforeWriteMsg=warning  WriteAfterWriteMsg=warning  WriteAfterReadMsg=warning  ShowAdditionalParam=off  OutDataTypeStr=int16
  Data Store Memory4 : DataStoreMemory  DataStoreName=Spe_Kp  ReadBeforeWriteMsg=warning  WriteAfterWriteMsg=warning  WriteAfterReadMsg=warning  ShowAdditionalParam=off  OutDataTypeStr=single
  Data Store Memory5 : DataStoreMemory  DataStoreName=Spe_Ki  ReadBeforeWriteMsg=warning  WriteAfterWriteMsg=warning  WriteAfterReadMsg=warning  ShowAdditionalParam=off  OutDataTypeStr=single
  Data Store Memory6 : DataStoreMemory  DataStoreName=W_I  ReadBeforeWriteMsg=warning  WriteAfterWriteMsg=warning  WriteAfterReadMsg=warning  ShowAdditionalParam=off  OutDataTypeStr=single
  Data Store Read1 : DataStoreRead  DataStoreName=W_P  DataStoreElements=W_P  IndexOptions=Index vector (dialog)  Indices=1  OutputSizes=1
  Data Store Read2 : DataStoreRead  DataStoreName=W_I  DataStoreElements=W_I  IndexOptions=Index vector (dialog)  Indices=1  OutputSizes=1
  Data Store Read3 : DataStoreRead  DataStoreName=Spe_Act  DataStoreElements=Spe_Act  IndexOptions=Index vector (dialog)  Indices=1  OutputSizes=1
  Data Store Read4 : DataStoreRead  DataStoreName=Spe_Kp  DataStoreElements=Spe_Kp  IndexOptions=Index vector (dialog)  Indices=1  OutputSizes=1
  Data Store Read5 : DataStoreRead  DataStoreName=Spe_Ki  DataStoreElements=Spe_Ki  IndexOptions=Index vector (dialog)  Indices=1  OutputSizes=1
  Data Store Write1 : DataStoreWrite  DataStoreName=Id_PIDcal  DataStoreElements=Id_PIDcal  IndexOptions=Index vector (dialog)  Indices=1  OutputSizes=1
  Gain : Gain  Gain=0.001
  Gain3 : Gain  Gain=1/6  OutDataTypeStr=single
  Inte_Sat : Saturate  UpperLimit=114  LowerLimit=-114
  Inte_Sat1 : Saturate  UpperLimit=114  LowerLimit=-114
  Inte_Switch : Switch  SaturateOnIntegerOverflow=off  InputSameDT=off
  Inte_sat_Lower : Switch  Criteria=u2 ~= 0  OutDataTypeStr=single  SaturateOnIntegerOverflow=off  InputSameDT=off
  Inte_sat_Upper : Switch  Criteria=u2 ~= 0  OutDataTypeStr=single  SaturateOnIntegerOverflow=off  InputSameDT=off
  LOWPASS : Subsystem  Commented=on
  Relational Operator : RelationalOperator  OutDataTypeStr=boolean  RndMeth=Simplest  InputSameDT=off
  Relational Operator1 : RelationalOperator  OutDataTypeStr=boolean  RndMeth=Simplest  InputSameDT=off
  Relational Operator2 : RelationalOperator  Operator===  OutDataTypeStr=boolean  RndMeth=Simplest  InputSameDT=off
  Relational Operator3 : RelationalOperator  Operator===  OutDataTypeStr=boolean  RndMeth=Simplest  InputSameDT=off
  SpeErr_by_I : Product  OutDataTypeStr=single
  SpeErr_by_P : Product  OutDataTypeStr=single
  Sum : Sum  Inputs=|++
  Sum1 : Sum  Inputs=-+|  OutDataTypeStr=single
  Sum3 : Sum  Inputs=|+-  OutDataTypeStr=single
  Sum4 : Sum  Inputs=|+-
  Switch : Switch  Criteria=u2 ~= 0  SaturateOnIntegerOverflow=off  InputSameDT=off
  Switch1 : Switch  Criteria=u2 ~= 0  SaturateOnIntegerOverflow=off  InputSameDT=off
  Switch2 : Switch  Criteria=u2 ~= 0  SaturateOnIntegerOverflow=off  InputSameDT=off
  Unit Delay : UnitDelay  SampleTime=-1  HasFrameUpgradeWarning=on
  WeakMagnetism : Subsystem
  Id_desired : Outport  VectorParamsAs1DForOutWhenUnconnected=off
  iq_desired : Outport  Port=2  VectorParamsAs1DForOutWhenUnconnected=off
  Iq_PIDcal : Outport  Port=3  VectorParamsAs1DForOutWhenUnconnected=off
  wires:
  Sum4/1 -> Accuracy_Ctrl1/2(errSpd), Accuracy_Ctrl/2(errSpd), SpeErr_by_P/1
  Data Store Read4/1 -> SpeErr_by_P/2
  Data Store Read5/1 -> SpeErr_by_I/2
  Inte_Sat/1 -> Switch2/1
  Gain3/1 -> Sum4/2
  Spe_Desired/1 -> Sum4/1, WeakMagnetism/2(Speed_desired)
  Add/1 -> Inte_Sat/1
  SpeErr_by_P/1 -> SpeErr_by_I/1, Accuracy_Ctrl/3(SPDpterm_in)
  SpeErr_by_I/1 -> Accuracy_Ctrl1/3(SPDiterm_in)
  Unit Delay/1 -> Switch/3
  Pressure_Cmplt/1 -> Accuracy_Ctrl1/1(Pressure_Cmplt), Accuracy_Ctrl/1(Pressure_Cmplt)
  Constant/1 -> Switch/1
  EHB_mode/1 -> Relational Operator2/1, Relational Operator3/1
  Constant1/1 -> Relational Operator2/2
  Relational Operator2/1 -> Switch1/2
  Constant2/1 -> Switch1/1
  Switch1/1 -> Id_desired/1, Data Store Write1/1
  WeakMagnetism/1(id_desired) -> Switch1/3
  Relational Operator3/1 -> Switch2/2
  Constant3/1 -> Relational Operator3/2
  Switch2/1 -> WeakMagnetism/1(Iq_closed_input)
  Constant4/1 -> Switch2/3
  Data Store Read1/1 -> WeakMagnetism/5(w_P)
  Data Store Read2/1 -> WeakMagnetism/6(w_I)
  Vd/1 -> WeakMagnetism/3(Vd)
  Vq/1 -> WeakMagnetism/4(Vq)
  Data Store Read3/1 -> Gain3/1
  EHB_Initiate/1 -> Switch/2, Accuracy_Ctrl1/4(EHB_Initiate), Accuracy_Ctrl/4(EHB_Initiate)
  Relational Operator1/1 -> Inte_sat_Lower/2
  Inte_sat_Upper/1 -> Inte_Switch/1
  Cur_Upper/1 -> Sum1/2, Relational Operator/2
  Sum/1 -> Inte_Sat1/1
  Cur_lower/1 -> Sum3/1, Relational Operator1/2
  Accuracy_Ctrl1/1(SPDiterm_out) -> Gain/1
  Inte_sat_Lower/1 -> Inte_Switch/3
  Sum1/1 -> Inte_sat_Upper/1
  Sum3/1 -> Inte_sat_Lower/3
  Accuracy_Ctrl/1(SPDpterm_out) -> Inte_Switch/2, Sum3/2, Relational Operator1/1, Relational Operator/1, Sum1/1, Add/1
  Gain/1 -> Sum/1
  Relational Operator/1 -> Inte_sat_Upper/2
  Switch/1 -> Sum/2
  Inte_Switch/1 -> Unit Delay/1, Add/2
  Inte_Sat1/1 -> Inte_sat_Upper/3, Inte_sat_Lower/1
  WeakMagnetism/2(iq_desired) -> Iq_PIDcal/1, iq_desired/1
